simulink model "Basics_9"  (R2018a)
settings: Solver=ode1  StartTime=0.0  StopTime=20  FixedStep=1e-4  RelTol=1e-3  EnableMultiTasking=on
settings Model: Creator=ayyrao  LastModifiedBy=ayyrao
settings DataIOCC: LimitDataPoints=on  SaveFormat=Array
settings OptimizationCC: LifeSpan=inf
settings DebuggingCC: SFUnexpectedBacktrackingDiag=warning  SFNoUnconditionalDefaultTransitionDiag=warning  SFExecutionAtInitializationDiag=none
settings HardwareCC: ProdBitPerPointer=32  ProdBitPerSizeT=32  ProdBitPerPtrDiffT=32  ProdLargestAtomicFloat=None  ProdIntDivRoundTo=Undefined  ProdEndianess=Unspecified  ProdWordSize=32  ProdHWDeviceType=32-bit Generic
settings ModelReferenceCC: PropagateSignalLabelsOutOfModel=off
settings CodeAppCC: StateflowObjectComments=on
settings GRTTargetCC: TargetLangStandard=C89/C90 (ANSI)  GeneratePreprocessorConditionals=Disable all
settings ConfigComp: CovMetricSettings=dw  CovHtmlReporting=on  CovSaveCumulativeToWorkspaceVar=on  CovSaveSingleToWorkspaceVar=on  CovExternalEMLEnable=off

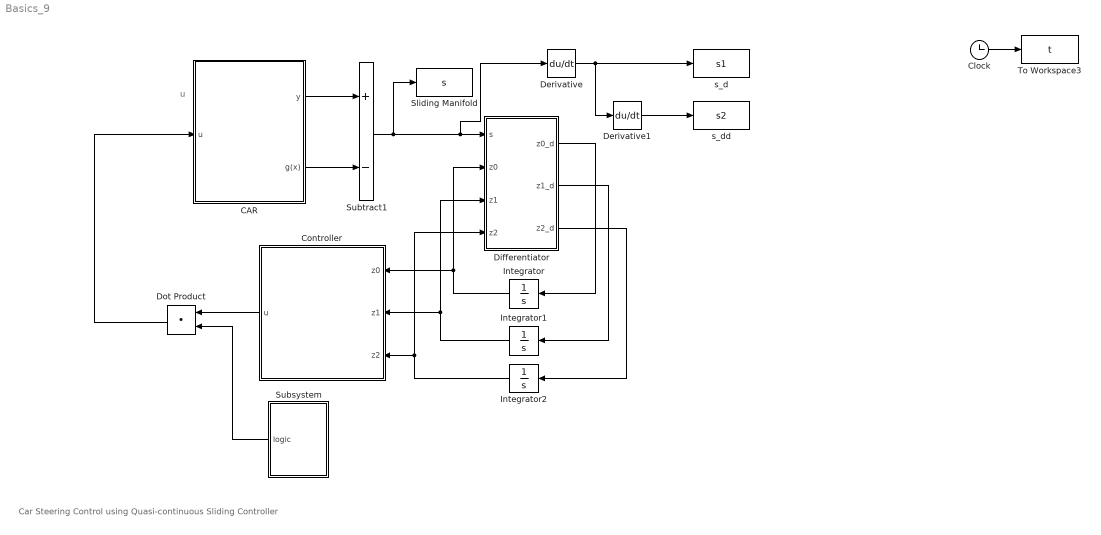
== system Basics_9 ==
  note: u
  note: Car Steering Control using Quasi-continuous Sliding Controller
  CAR : Subsystem
      mask Display: image('bmw-3-series-modellfinder.png');
  Clock : Clock
  Controller : MATLAB Function  TreatAsAtomicUnit=on
  Derivative : Derivative
  Derivative1 : Derivative
  Differentiator : MATLAB Function  TreatAsAtomicUnit=on
  Dot Product : DotProduct  InputSameDT=on  OutDataTypeStr=Inherit: Inherit via internal rule
  Integrator : Integrator
  Integrator1 : Integrator
  Integrator2 : Integrator
  Sliding Manifold : ToWorkspace  VariableName=s  SampleTime=-1
  Subsystem : Subsystem
  Subtract1 : Sum  Inputs=+-
  To Workspace3 : ToWorkspace  VariableName=t  SampleTime=-1
  s_d : ToWorkspace  VariableName=s1  SampleTime=-1
  s_dd : ToWorkspace  VariableName=s2  SampleTime=-1
  wires:
  Clock/1 -> To Workspace3/1
  CAR/1(y) -> Subtract1/1
  CAR/2(g(x)) -> Subtract1/2
  Subtract1/1 -> Derivative/1, Differentiator/1(s), Sliding Manifold/1
  Differentiator/1(z0_d) -> Integrator/1
  Integrator/1 -> Controller/1(z0), Differentiator/2(z0)
  Differentiator/2(z1_d) -> Integrator1/1
  Integrator1/1 -> Controller/2(z1), Differentiator/3(z1)
  Differentiator/3(z2_d) -> Integrator2/1
  Integrator2/1 -> Controller/3(z2), Differentiator/4(z2)
  Derivative/1 -> Derivative1/1, s_d/1
  Derivative1/1 -> s_dd/1
  Dot Product/1 -> CAR/1(u)
  Subsystem/1(logic) -> Dot Product/2
  Controller/1(u) -> Dot Product/1

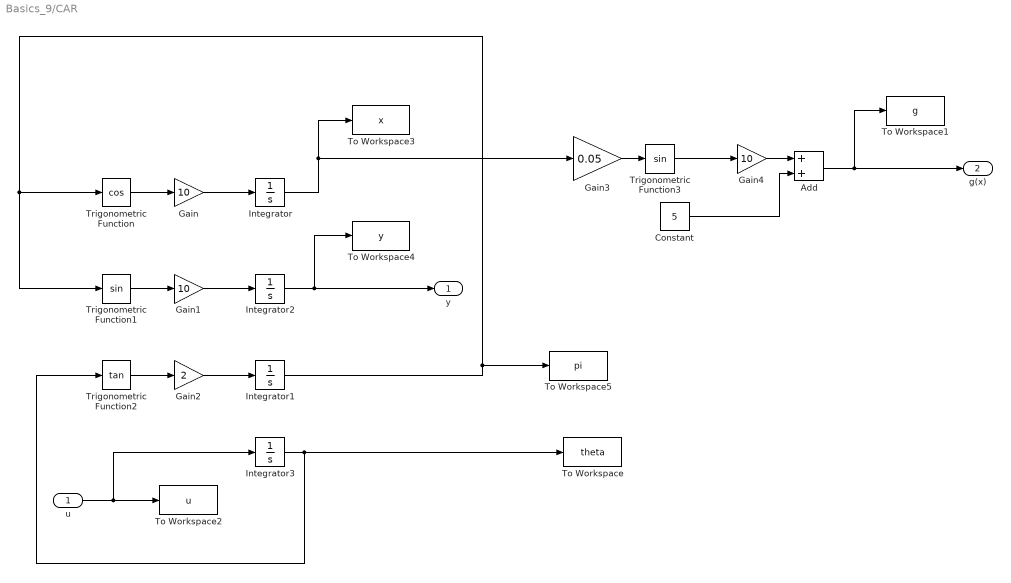
== system Basics_9/CAR ==
  u : Inport
  Add : Sum
  Constant : Constant  Value=5
  Gain : Gain  Gain=10
  Gain1 : Gain  Gain=10
  Gain2 : Gain  Gain=2
  Gain3 : Gain  Gain=0.05
  Gain4 : Gain  Gain=10
  Integrator{,1..3} (4 alike) : Integrator
  To Workspace : ToWorkspace  VariableName=theta  SampleTime=-1
  To Workspace1 : ToWorkspace  VariableName=g  SampleTime=-1
  To Workspace2 : ToWorkspace  VariableName=u  SampleTime=-1
  To Workspace3 : ToWorkspace  VariableName=x  SampleTime=-1
  To Workspace4 : ToWorkspace  VariableName=y  SampleTime=-1
  To Workspace5 : ToWorkspace  VariableName=pi  SampleTime=-1
  Trigonometric Function : Trigonometry  Operator=cos
  Trigonometric Function1 : Trigonometry
  Trigonometric Function2 : Trigonometry  Operator=tan
  Trigonometric Function3 : Trigonometry
  y : Outport
  g(x) : Outport  Port=2
  wires:
  u/1 -> Integrator3/1, To Workspace2/1
  Gain/1 -> Integrator/1
  Trigonometric Function/1 -> Gain/1
  Trigonometric Function1/1 -> Gain1/1
  Gain1/1 -> Integrator2/1
  Trigonometric Function2/1 -> Gain2/1
  Gain2/1 -> Integrator1/1
  Integrator1/1 -> To Workspace5/1, Trigonometric Function1/1, Trigonometric Function/1
  Integrator3/1 -> Trigonometric Function2/1, To Workspace/1
  Gain3/1 -> Trigonometric Function3/1
  Trigonometric Function3/1 -> Gain4/1
  Gain4/1 -> Add/1
  Constant/1 -> Add/2
  Integrator/1 -> Gain3/1, To Workspace3/1
  Integrator2/1 -> y/1, To Workspace4/1
  Add/1 -> g(x)/1, To Workspace1/1

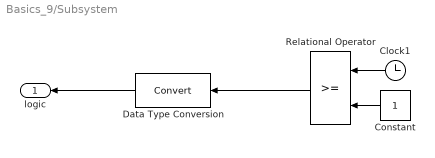
== system Basics_9/Subsystem ==
  Clock1 : Clock
  Constant : Constant
  Data Type Conversion : DataTypeConversion
  Relational Operator : RelationalOperator  OutDataTypeStr=boolean  RndMeth=Simplest
  logic : Outport
  wires:
  Clock1/1 -> Relational Operator/1
  Constant/1 -> Relational Operator/2
  Relational Operator/1 -> Data Type Conversion/1
  Data Type Conversion/1 -> logic/1

== matlab function Basics_9/Differentiator ==
  data: s input; z0 input; z1 input; z2 input; z0_d output; z1_d output; z2_d output
function [z0_d,z1_d,z2_d]= fcn(s,z0,z1,z2)
%%% JKD Power and Energy solutions
%% Differentiator
v0 = -14.7361*(abs(z0-s))^(2/3)*sign(z0-s)+z1;
v1 = -30*(abs(z1-v0))^(1/2)*sign(z1-v0)+z2;
z0_d = v0;
z1_d  = v1;
z2_d  = -400*sign(z2-v1);
end

== matlab function Basics_9/Controller ==
  data: z0 input; z1 input; z2 input; u output
function u= fcn1(z0,z1,z2)
%%% JKD Power and Energy solutions
%% Quasi-continuous Sliding controller
u = -(z2+2*((abs(z1)+(abs(z0))^(2/3))^(-1/2))*(z1+(abs(z0))^(2/3)*sign(z0)))/(abs(z2)+2*((abs(z1)+(abs(z0))^(2/3))^(1/2)));
if isnan(u)
    u=0;
end
end
